simulink model "lorenz_sol"  (R2023b)
settings: Solver=ode3  StartTime=0.0  StopTime=100  FixedStep=1e-3  RelTol=1e-3
settings Model: Creator=jerome  LastModifiedBy=jerome

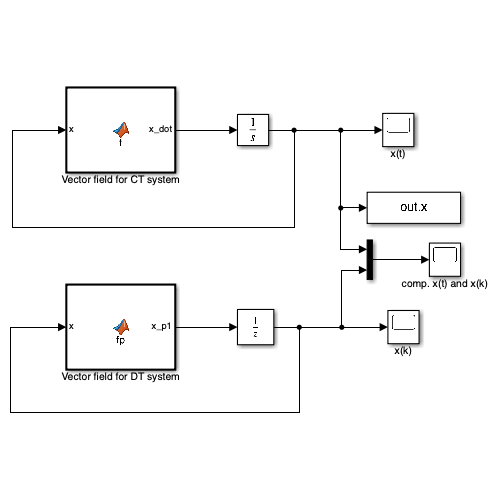
[thumbnail: Simulink's stored preview of the top-level diagram]
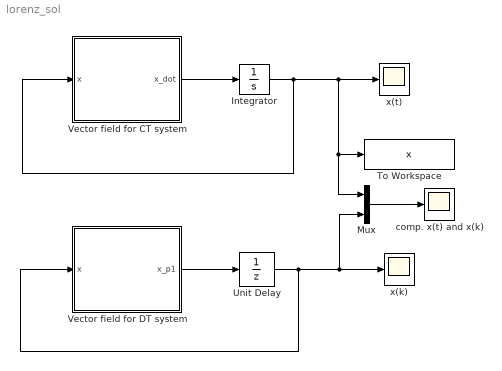
== system lorenz_sol ==
  Integrator : Integrator  InitialCondition=[0;1;0]
  Mux : Mux  Inputs=2
  To Workspace : ToWorkspace  VariableName=x  SampleTime=-1
  Unit Delay : UnitDelay  InitialCondition=[0;1;0]  SampleTime=1e-3  HasFrameUpgradeWarning=on
  Vector field for CT system : MATLAB Function  TreatAsAtomicUnit=on
  Vector field for DT system : MATLAB Function  TreatAsAtomicUnit=on
  comp. x(t) and x(k) : Scope
  x(k) : Scope
  x(t) : Scope
  wires:
  Vector field for CT system/1(x_dot) -> Integrator/1
  Integrator/1 -> x(t)/1, Mux/1, To Workspace/1, Vector field for CT system/1(x)
  Vector field for DT system/1(x_p1) -> Unit Delay/1
  Unit Delay/1 -> Mux/2, x(k)/1, Vector field for DT system/1(x)
  Mux/1 -> comp. x(t) and x(k)/1

== matlab function lorenz_sol/Vector field for CT system ==
  data: x input; x_dot output
function x_dot = f(x) % nonlinear mapping

rho = 28;
sigma = 10;
beta = 8/3;

x_dot = [ sigma*(x(2) - x(1))  ;
          x(1)*(rho-x(3))-x(2) ; 
          x(1)*x(2)-beta*x(3) ];

== matlab function lorenz_sol/Vector field for DT system ==
  data: x input; x_p1 output
function x_p1 = fp(x) % nonlinear mapping f "prime" (discrete-time)
% x_p1 means x(k+1)
rho = 28;
sigma = 10;
beta = 8/3;

Ts = 1e-3; % sampling time

x_p1 = x + Ts*[ sigma*(x(2) - x(1))  ;
                x(1)*(rho-x(3))-x(2) ; 
                x(1)*x(2)-beta*x(3) ];
